simulink model "lab1d"  (R2022b)
settings: Solver=FixedStepAuto  StartTime=0.0  StopTime=65  FixedStep=1/512  RelTol=1e-3
libraries: dsparch4 x1
settings Model: Creator=simja  LastModifiedBy=simja
settings SolverCC: AutoInsertRateTranBlk=on
settings DataIOCC: ReturnWorkspaceOutputs=off

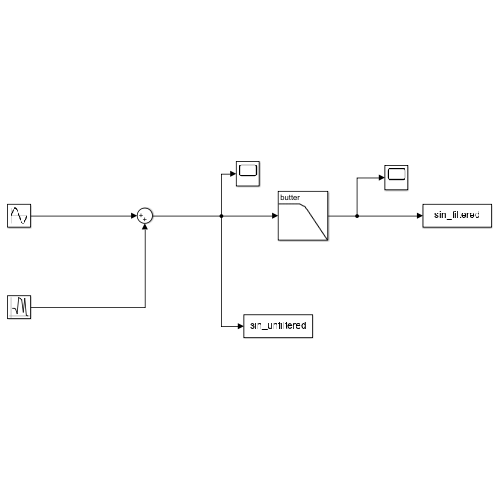
[thumbnail: Simulink's stored preview of the top-level diagram]
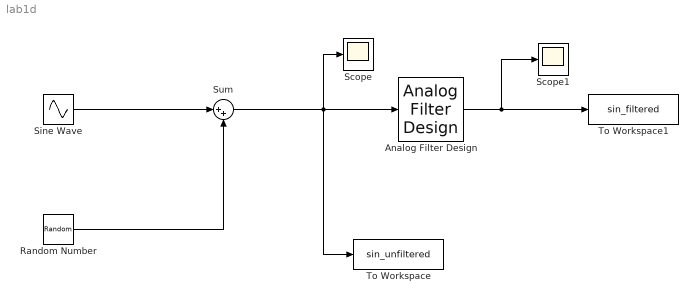
== system lab1d ==
  Analog Filter Design : dsparch4/Analog Filter Design  method=Butterworth  filttype=Lowpass  N=3  Wlo=23*2*pi  Whi=80  Rp=2  Rs=40
  Random Number : RandomNumber  Variance=0.005
  Scope : Scope
  Scope1 : Scope
  Sine Wave : Sin  Amplitude=0.1  Frequency=2*pi*7  SampleTime=0
  Sum : Sum  Inputs=|++
  To Workspace : ToWorkspace  VariableName=sin_unfiltered  SaveFormat=Structure With Time  SampleTime=-1
  To Workspace1 : ToWorkspace  VariableName=sin_filtered  SaveFormat=Structure With Time  SampleTime=-1
  wires:
  Sine Wave/1 -> Sum/1
  Random Number/1 -> Sum/2
  Sum/1 -> To Workspace/1, Analog Filter Design/1, Scope/1
  Analog Filter Design/1 -> To Workspace1/1, Scope1/1
